simulink model "dynamics"  (R2018a)
settings: Solver=VariableStepAuto  StartTime=0.0  StopTime=100.0  RelTol=1e-3
InitFcn:
  | param
undefined symbols (not defined in the file or in its folder): P
libraries: simulink x2
settings Model: Creator=mark  LastModifiedBy=mark

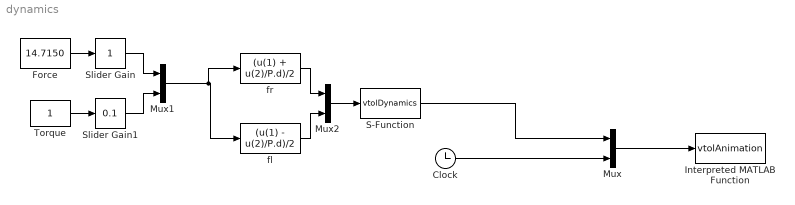
== system dynamics ==
  Clock : Clock
  Force : Constant  Value=14.7150
  Interpreted MATLAB Function : MATLABFcn  MATLABFcn=vtolAnimation  OutputDimensions=0
  Mux : Mux  Inputs=2
  Mux1 : Mux  Inputs=2
  Mux2 : Mux  Inputs=2
  S-Function : S-Function  FunctionName=vtolDynamics  Parameters=P  SFunctionDeploymentMode=off  EnableBusSupport=off
  Slider Gain : simulink/Math Operations/Slider Gain  gain=1  low=0  high=2
  Slider Gain1 : simulink/Math Operations/Slider Gain  gain=0.1  low=0  high=2
  Torque : Constant
  fl : Fcn  Expr=(u(1) - u(2)/P.d)/2
  fr : Fcn  Expr=(u(1) + u(2)/P.d)/2
  wires:
  Mux/1 -> Interpreted MATLAB Function/1
  Clock/1 -> Mux/2
  S-Function/1 -> Mux/1
  Torque/1 -> Slider Gain1/1
  Force/1 -> Slider Gain/1
  Slider Gain/1 -> Mux1/1
  Slider Gain1/1 -> Mux1/2
  Mux1/1 -> fr/1, fl/1
  fl/1 -> Mux2/2
  fr/1 -> Mux2/1
  Mux2/1 -> S-Function/1
